simulink model "tricopter_simulation"  (Simulink 7.8)
settings: Solver=FixedStepDiscrete  StartTime=0.0  StopTime=10  FixedStep=dt_sim  RelTol=1e-3
InitFcn:
  | Init
values from neighbouring files (symbols this model uses):
  act_latency = 1*dt_sim    (= 0.005)    [Init.m]
  D = 1    [Init.m]
  dt_sim = 0.005    [Init.m]
  gvec = [0 0 9.81]'    [Init.m]
  J = diag([0.25*m*(D/2)^2 0.25*m*(D/2)^2 0.5*m*(D/2)^2])    [Init.m]
  k = 0.0000192    (= 1.92e-05)    [Init.m]
  L = 0.5    [Init.m]
  m = 1    [Init.m]
  max_rpm = 7000*pi/30    (= 733.038285838)    [Init.m]
  min_rpm = 0    [Init.m]
  rho = 1.26    [Init.m]
undefined symbols (not defined in the file or in its folder): DiscIntNeverNeededParam, waitfortreal
libraries: animation_lib x1, simulink x1
(part 1 of 2)
settings Model: Creator=sven  LastModifiedBy=sven  BufferReuse=off
settings DataIOCC: LimitDataPoints=off  SaveOutput=off  SignalLogging=off  DSMLogging=off  SaveTime=off  SignalLoggingName=sigsOut
settings OptimizationCC: InlineParams=on  BufferReuse=off  InitFltsAndDblsToZero=on
settings DebuggingCC: ConsistencyChecking=error  SignalInfNanChecking=error  SignalRangeChecking=error  ReadBeforeWriteMsg=DisableAll  WriteAfterWriteMsg=DisableAll  WriteAfterReadMsg=DisableAll  AlgebraicLoopMsg=error  ArtificialAlgebraicLoopMsg=error  SaveWithDisabledLinksMsg=error  SaveWithParameterizedLinksMsg=error  UnderspecifiedInitializationDetection=Simplified  MergeDetectMultiDrivingBlocksExec=error  BlockPriorityViolationMsg=error  MinStepSizeMsg=error  TimeAdjustmentMsg=warning  SolverPrmCheckMsg=error  InheritedTsInSrcMsg=error  DiscreteInheritContinuousMsg=error  SingleTaskRateTransMsg=error  TasksWithSamePriorityMsg=error  SigSpecEnsureSampleTimeMsg=error  CheckMatrixSingularityMsg=error  IntegerOverflowMsg=error  ParameterUnderflowMsg=error  ParameterPrecisionLossMsg=error  ParameterTunabilityLossMsg=error  FixptConstUnderflowMsg=error  FixptConstOverflowMsg=error  FixptConstPrecisionLossMsg=error  UnderSpecifiedDataTypeMsg=error  SignalLabelMismatchMsg=error  UnconnectedInputMsg=error  UnconnectedOutputMsg=error  UnconnectedLineMsg=error  SFcnCompatibilityMsg=warning  UniqueDataStoreMsg=error  BusObjectLabelMismatch=error  RootOutportRequireBusObject=error  AssertControl=EnableAll  ModelReferenceIOMsg=error  ModelReferenceVersionMismatchMessage=error  ModelReferenceIOMismatchMessage=error  ModelReferenceCSMismatchMessage=error  UnknownTsInhSupMsg=error  ModelReferenceDataLoggingMessage=error  SimStateInterfaceChecksumMismatchMsg=error  StrictBusMsg=ErrorOnBusTreatedAsVector  BusNameAdapt=ErrorWithoutRepair  NonBusSignalsTreatedAsBus=error  SFUnusedDataAndEventsDiag=error  SFUnexpectedBacktrackingDiag=error  SFInvalidInputDataAccessInChartInitDiag=error  SFNoUnconditionalDefaultTransitionDiag=error  SFTransitionOutsideNaturalParentDiag=error
settings HardwareCC: TargetUnknown=on
settings RTWCC: IncludeERTFirstTime=on
settings GRTTargetCC: TargetFcnLib=ansi_tfl_tmw.mat

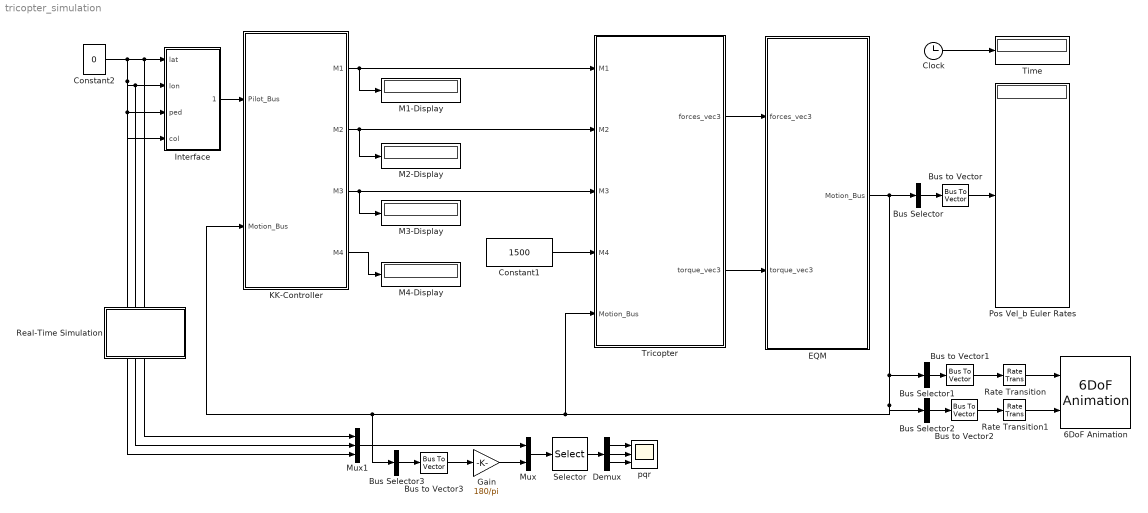
== system tricopter_simulation ==
  6DoF Animation : animation_lib/6DoF Animation  u1=[0 40 -20 20 -50 -30]  u2=0.1  u3=1.0  u4=[40 0 -50]  u5=Fixed position  u6=[20 5 -31]  u7=10  u8=on
  Bus Selector : BusSelector  OutputSignals=pos.x,pos.y,pos.z,vel_body.ub,vel_body.vb,vel_body.wb,attitude.phi,attitude.theta,attitude.psi,rate.p,rate.q,rate.r  OutputAsBus=on
  Bus Selector1 : BusSelector  OutputSignals=pos.x,pos.y,pos.z  OutputAsBus=on
  Bus Selector2 : BusSelector  OutputSignals=attitude.phi,attitude.theta,attitude.psi  OutputAsBus=on
  Bus Selector3 : BusSelector  OutputSignals=rate.p,rate.q,rate.r  OutputAsBus=on
  Bus to Vector{,1..3} (4 alike) : BusToVector
  Clock : Clock
  Constant1 : Constant  Value=1500
  Constant2 : Constant  Value=0
  Demux : Demux  Outputs=3
  EQM : Subsystem
  Gain : Gain  Gain=180/pi
  Interface : Subsystem
  KK-Controller : Subsystem
  M1-Display : Display
  M2-Display : Display
  M3-Display : Display
  M4-Display : Display
  Mux : Mux  Inputs=2
  Mux1 : Mux  Inputs=3
  Pos Vel_b Euler Rates : Display
  Rate Transition : RateTransition  OutPortSampleTime=0.2
  Rate Transition1 : RateTransition  OutPortSampleTime=0.2
  Real-Time Simulation : Subsystem
      mask Display: disp('SL RT')
  Selector : Selector  InputPortWidth=6  IndexOptions=Index vector (dialog)  Indices=[1 4 2 5 3 6]  OutputSizes=1
  Time : Display
  Tricopter : Subsystem
  pqr : Scope  NumInputPorts=3
      settings: YMin=-5~-4~-5  YMax=10~0~5
  wires:
  Tricopter/2(torque_vec3) -> EQM/2(torque_vec3)
  Tricopter/1(forces_vec3) -> EQM/1(forces_vec3)
  EQM/1(Motion_Bus) -> Bus Selector/1, Bus Selector1/1, Tricopter/5(Motion_Bus), KK-Controller/2(Motion_Bus), Bus Selector3/1, Bus Selector2/1
  Constant1/1 -> Tricopter/4(M4)
  KK-Controller/1(M1) -> M1-Display/1, Tricopter/1(M1)
  KK-Controller/2(M2) -> M2-Display/1, Tricopter/2(M2)
  KK-Controller/3(M3) -> M3-Display/1, Tricopter/3(M3)
  Interface/1(Pilot_Bus) -> KK-Controller/1(Pilot_Bus)
  KK-Controller/4(M4) -> M4-Display/1
  Bus Selector/1 -> Bus to Vector/1
  Bus to Vector/1 -> Pos Vel_b Euler Rates/1
  Clock/1 -> Time/1
  Constant2/1 -> Interface/3(ped), Interface/4(col), Mux1/3, Interface/2(lon), Mux1/2, Interface/1(lat), Mux1/1
  Bus Selector1/1 -> Bus to Vector1/1
  Bus Selector2/1 -> Bus to Vector2/1
  Bus to Vector1/1 -> Rate Transition/1
  Bus to Vector2/1 -> Rate Transition1/1
  Rate Transition/1 -> 6DoF Animation/1
  Rate Transition1/1 -> 6DoF Animation/2
  Mux/1 -> Selector/1
  Bus Selector3/1 -> Bus to Vector3/1
  Gain/1 -> Mux/2
  Mux1/1 -> Mux/1
  Selector/1 -> Demux/1
  Demux/1 -> pqr/1
  Demux/2 -> pqr/2
  Demux/3 -> pqr/3
  Bus to Vector3/1 -> Gain/1

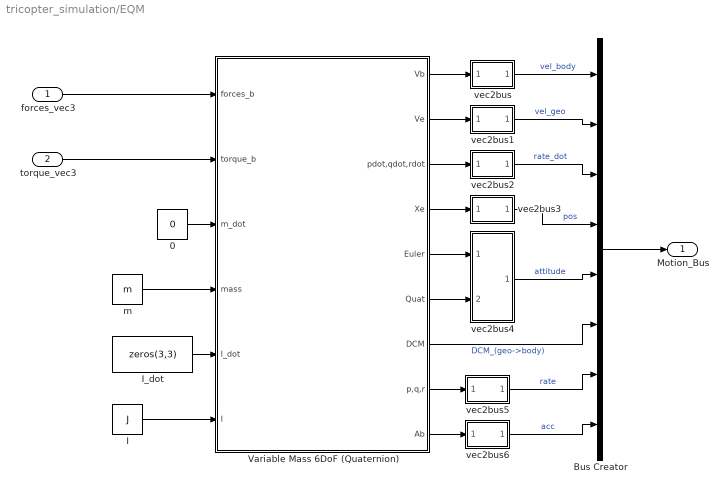
== system tricopter_simulation/EQM ==
  forces_vec3 : Inport
  torque_vec3 : Inport  Port=2
  0 : Constant  Value=0
  Bus Creator : BusCreator  Inputs=8
  I : Constant  Value=J
  I_dot : Constant  Value=zeros(3,3)
  Variable Mass 6DoF (Quaternion) : Subsystem  mask{xme_0=[0 0 0], Vm_0=[0 0 0], eul_0=[0 0 0], pm_0=[10 0 0]*pi/180, dt_sim=dt_sim, run_translation=off}
      mask prompts: xme_0 "Inertial position in inertial axes [Xe, Ye Ze]"; Vm_0 "Inertial velocity in body axes [u, v, w]"; eul_0 "Inertial Euler orientation [roll, pitch, yaw]"; pm_0 "Inertial body rotation rates[p, q, r]"; dt_sim "Sample Time"; run_translation "Run Translational Motion"
      mask help:
      | Variable Mass 6DoF (Quaternion)
      | (rebuild from MATLAB AeroSpace Blockset)
      mask Help:
      | Inputs and Outputs
      | 
      | The first input to the block is a vector containing the three applied forces.
      | The second input is a vector containing the three applied moments.
      | The third input is a scalar containing the rate of change of mass.
      | The fourth input is a scalar containing the mass
      | The fifth input is a 3-by-3 matrix for the rate of change of inertia tensor matrix.
      | The sixth input is a 3-by-3 matrix for the inertia tensor matrix.
      | 
      | The first output is a three-element vector containing the velocity in the Earth-fixed reference frame.
      | The second output is a three-element vector containing the position in the Earth-fixed reference frame.
      | The third output is a three-element vector containing the Euler rotation angles [roll, pitch, yaw], in radians.
      | The fourth output is a 3-by-3 matrix for the coordinate transformation from Earth-fixed axes to body-fixed axes.
      | The fifth output is a three-element vector containing the velocity in the body-fixed frame.
      | The sixth output is a three-element vector containing the angular rates in body-fixed axes, in radians per second.
      | The seventh output is a three-element vector containing the angular accelerations in body-fixed axes, in radians per second. The eighth output is a three-element vector containing the accelerations in body-fixed axes.
      mask Display:
      | port_label('input',1,'Fb_xyz (N)')
      | port_label('input',2,'Mb_xyz (Nm)')
      | port_label('input',3,'dm/dt (kg/s)')
      | port_label('input',4,'m (kg)')
      | port_label('input',5,'dI/dt (kgm^2/s)')
      | port_label('input',6,'I (kgm^2)')
      | port_label('output',1,'Vb (m/s)')
      | port_label('output',2,'Ve (m/s)')
      | port_label('output',3,'pqrdot')
      | port_label('output',4,'Xe')
      | port_label('output',5,'phi theta psi (rad)')
      | port_label('output',6,'quaternions')
      | port_label('output',7,'DCM')
      | port_label('output',8,'pqr')
      | port_label('output',9,'Ab (m/s^2)')
  m : Constant  Value=m
  vec2bus : Subsystem
  vec2bus1 : Subsystem
  vec2bus2 : Subsystem
  vec2bus3 : Subsystem
  vec2bus4 : Subsystem
  vec2bus5 : Subsystem
  vec2bus6 : Subsystem
  Motion_Bus : Outport
  wires:
  vec2bus6/1(bus) -> Bus Creator/8  "acc"
  vec2bus5/1(bus) -> Bus Creator/7  "rate"
  Variable Mass 6DoF (Quaternion)/7(DCM) -> Bus Creator/6  "DCM_(geo->body)"
  vec2bus4/1(bus) -> Bus Creator/5  "attitude"
  vec2bus3/1(bus) -> Bus Creator/4  "pos"
  vec2bus2/1(bus) -> Bus Creator/3  "rate_dot"
  vec2bus1/1(bus) -> Bus Creator/2  "vel_geo"
  vec2bus/1(bus) -> Bus Creator/1  "vel_body"
  Variable Mass 6DoF (Quaternion)/6(Quat) -> vec2bus4/2(quat)
  Variable Mass 6DoF (Quaternion)/9(Ab) -> vec2bus6/1(vec)
  Variable Mass 6DoF (Quaternion)/8(p,q,r) -> vec2bus5/1(vec)
  Variable Mass 6DoF (Quaternion)/5(Euler) -> vec2bus4/1(euler)
  Variable Mass 6DoF (Quaternion)/4(Xe) -> vec2bus3/1(vec)
  Variable Mass 6DoF (Quaternion)/3(pdot,qdot,rdot) -> vec2bus2/1(vec)
  Variable Mass 6DoF (Quaternion)/2(Ve) -> vec2bus1/1(vec)
  Variable Mass 6DoF (Quaternion)/1(Vb) -> vec2bus/1(vec)
  I/1 -> Variable Mass 6DoF (Quaternion)/6(I)
  I_dot/1 -> Variable Mass 6DoF (Quaternion)/5(I_dot)
  m/1 -> Variable Mass 6DoF (Quaternion)/4(mass)
  0/1 -> Variable Mass 6DoF (Quaternion)/3(m_dot)
  forces_vec3/1 -> Variable Mass 6DoF (Quaternion)/1(forces_b)
  torque_vec3/1 -> Variable Mass 6DoF (Quaternion)/2(torque_b)
  Bus Creator/1 -> Motion_Bus/1

== system tricopter_simulation/Interface ==
  lat : Inport
  lon : Inport  Port=2
  ped : Inport  Port=3
  col : Inport  Port=4
  Bus Creator : BusCreator
  Constant1 : Constant  Value=1500
  Demux : Demux
  Display : Display
  Gain1 : Gain  Gain=-1  Multiplication=Matrix(K*u)  SaturateOnIntegerOverflow=on  OutDataTypeStr=Inherit: Same as input  ParamDataTypeStr=Inherit: Same as input
  Gain2 : Gain  Gain=500  Multiplication=Matrix(K*u)  SaturateOnIntegerOverflow=on  OutDataTypeStr=Inherit: Same as input  ParamDataTypeStr=Inherit: Same as input
  Mux2 : Mux
  Sum1 : Sum  SaturateOnIntegerOverflow=on
  Pilot_Bus : Outport
  wires:
  Mux2/1 -> Gain2/1
  lat/1 -> Mux2/1
  lon/1 -> Mux2/2
  ped/1 -> Mux2/3
  col/1 -> Gain1/1
  Constant1/1 -> Sum1/2
  Gain2/1 -> Sum1/1
  Gain1/1 -> Mux2/4
  Sum1/1 -> Demux/1, Display/1
  Demux/1 -> Bus Creator/1  "lat_us"
  Demux/2 -> Bus Creator/2  "lon_us"
  Demux/3 -> Bus Creator/3  "ped_us"
  Demux/4 -> Bus Creator/4  "col_us"
  Bus Creator/1 -> Pilot_Bus/1  "Pilot"

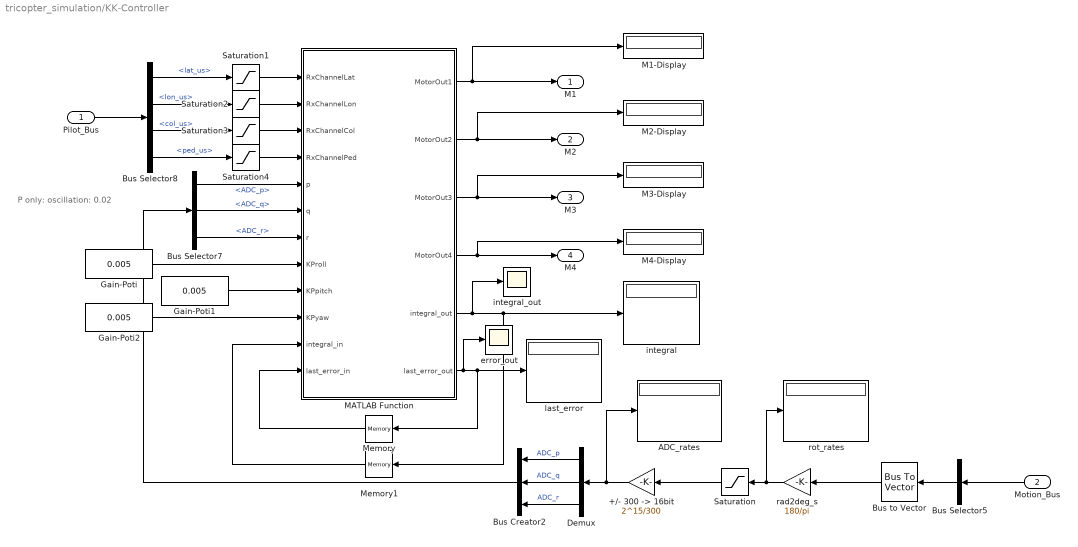
== system tricopter_simulation/KK-Controller ==
  note: P only: oscillation: 0.02
  Pilot_Bus : Inport
  Motion_Bus : Inport  Port=2
  "+/- 300 -> 16bit" : Gain  Gain=2^15/300
  ADC_rates : Display
  Bus Creator2 : BusCreator  Inputs=3
  Bus Selector5 : BusSelector  OutputSignals=rate.p,rate.q,rate.r  OutputAsBus=on
  Bus Selector7 : BusSelector  OutputSignals=ADC_p,ADC_q,ADC_r
  Bus Selector8 : BusSelector  OutputSignals=lat_us,lon_us,col_us,ped_us
  Bus to Vector : BusToVector
  Demux : Demux  Outputs=3
  Gain-Poti : Constant  Value=0.005
  Gain-Poti1 : Constant  Value=0.005
  Gain-Poti2 : Constant  Value=0.005
  M1-Display : Display
  M2-Display : Display
  M3-Display : Display
  M4-Display : Display
  MATLAB Function : MATLAB Function  TreatAsAtomicUnit=on
  Memory : Memory
  Memory1 : Memory
  Saturation : Saturate  UpperLimit=300  LowerLimit=-300
  Saturation{1..4} (4 alike) : Saturate  UpperLimit=2000  LowerLimit=1000
  error_out : Scope
      settings: YMin=-5.5  YMax=1  SaveName=ScopeData3
  integral : Display
  integral_out : Scope
      settings: TimeRange=10  YMin=-50  YMax=50  SaveName=ScopeData2
  last_error : Display
  rad2deg_s : Gain  Gain=180/pi
  rot_rates : Display
  M1 : Outport
  M2 : Outport  Port=2
  M3 : Outport  Port=3
  M4 : Outport  Port=4
  wires:
  MATLAB Function/1(MotorOut1) -> M1-Display/1, M1/1
  MATLAB Function/2(MotorOut2) -> M2-Display/1, M2/1
  MATLAB Function/3(MotorOut3) -> M3-Display/1, M3/1
  Bus Selector5/1 -> Bus to Vector/1
  rad2deg_s/1 -> Saturation/1, rot_rates/1
  Saturation/1 -> "+/- 300 -> 16bit"/1
  "+/- 300 -> 16bit"/1 -> Demux/1, ADC_rates/1
  Demux/1 -> Bus Creator2/1  "ADC_p"
  Demux/2 -> Bus Creator2/2  "ADC_q"
  Demux/3 -> Bus Creator2/3  "ADC_r"
  Bus Creator2/1 -> Bus Selector7/1
  Bus Selector7/1 -> MATLAB Function/5(p)  "<ADC_p>"
  Bus Selector7/2 -> MATLAB Function/6(q)  "<ADC_q>"
  Bus Selector7/3 -> MATLAB Function/7(r)  "<ADC_r>"
  MATLAB Function/4(MotorOut4) -> M4-Display/1, M4/1
  Bus to Vector/1 -> rad2deg_s/1
  Bus Selector8/1 -> Saturation1/1  "<lat_us>"
  Bus Selector8/2 -> Saturation2/1  "<lon_us>"
  Bus Selector8/3 -> Saturation3/1  "<col_us>"
  Bus Selector8/4 -> Saturation4/1  "<ped_us>"
  Saturation1/1 -> MATLAB Function/1(RxChannelLat)
  Saturation2/1 -> MATLAB Function/2(RxChannelLon)
  Saturation3/1 -> MATLAB Function/3(RxChannelCol)
  Saturation4/1 -> MATLAB Function/4(RxChannelPed)
  MATLAB Function/6(last_error_out) -> last_error/1, Memory/1, error_out/1
  MATLAB Function/5(integral_out) -> integral/1, Memory1/1, integral_out/1
  Memory/1 -> MATLAB Function/12(last_error_in)
  Memory1/1 -> MATLAB Function/11(integral_in)
  Motion_Bus/1 -> Bus Selector5/1
  Pilot_Bus/1 -> Bus Selector8/1
  Gain-Poti/1 -> MATLAB Function/8(KProll)
  Gain-Poti1/1 -> MATLAB Function/9(KPpitch)
  Gain-Poti2/1 -> MATLAB Function/10(KPyaw)

== system tricopter_simulation/Real-Time Simulation ==
  Clock : Clock
  MATLAB Fcn : MATLABFcn  MATLABFcn=waitfortreal(u)  OutputDimensions=0
  wires:
  Clock/1 -> MATLAB Fcn/1

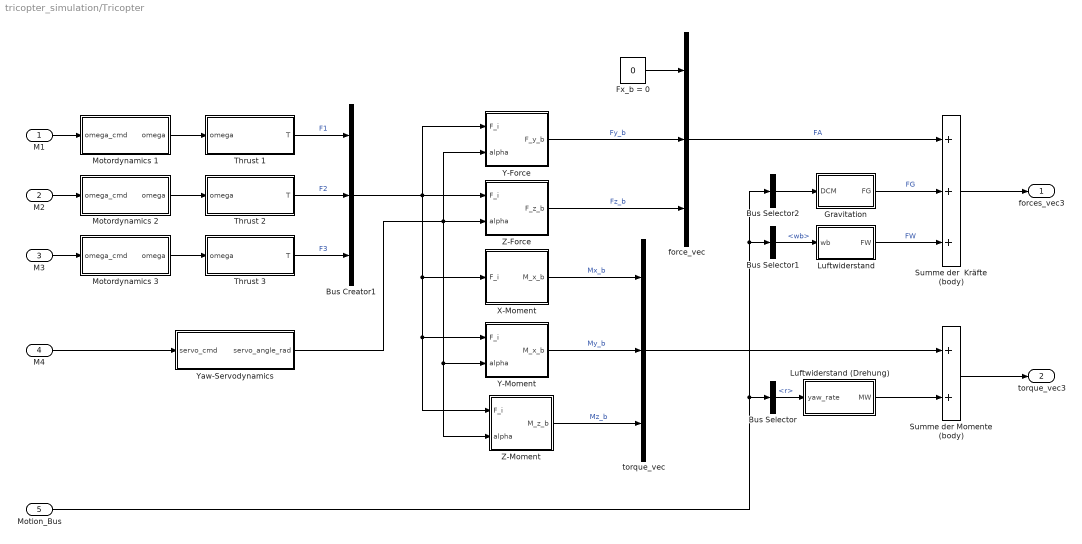
== system tricopter_simulation/Tricopter ==
  M1 : Inport
  M2 : Inport  Port=2
  M3 : Inport  Port=3
  M4 : Inport  Port=4
  Motion_Bus : Inport  Port=5
  Bus Creator1 : BusCreator  Inputs=3
  Bus Selector : BusSelector  OutputSignals=rate.r
  Bus Selector1 : BusSelector  OutputSignals=vel_body.wb
  Bus Selector2 : BusSelector  OutputSignals=DCM_(geo->body)  OutputAsBus=on
  Fx_b = 0 : Constant  Value=0
  Gravitation : Subsystem
  Luftwiderstand : Subsystem
  Luftwiderstand (Drehung) : Subsystem
  Motordynamics 1 : Subsystem
  Motordynamics 2 : Subsystem
  Motordynamics 3 : Subsystem
  Summe der  Kräfte (body) : Sum  Inputs=+++  SaturateOnIntegerOverflow=on
  Summe der Momente (body) : Sum  SaturateOnIntegerOverflow=on
  Thrust 1 : Subsystem
  Thrust 2 : Subsystem
  Thrust 3 : Subsystem
  X-Moment : Subsystem
  Y-Force : Subsystem
  Y-Moment : Subsystem
  Yaw-Servodynamics : Subsystem
  Z-Force : Subsystem
  Z-Moment : Subsystem
  force_vec : Mux  Inputs=3
  torque_vec : Mux  Inputs=3
  forces_vec3 : Outport
  torque_vec3 : Outport  Port=2
  wires:
  Motordynamics 1/1(omega) -> Thrust 1/1(omega)
  Summe der Momente (body)/1 -> torque_vec3/1
  Summe der  Kräfte (body)/1 -> forces_vec3/1
  Bus Selector2/1 -> Gravitation/1(DCM)
  Bus Selector1/1 -> Luftwiderstand/1(wb)  "<wb>"
  Bus Selector/1 -> Luftwiderstand (Drehung)/1(yaw_rate)  "<r>"
  Z-Moment/1(M_z_b) -> torque_vec/3  "Mz_b"
  Luftwiderstand (Drehung)/1(MW) -> Summe der Momente (body)/2
  torque_vec/1 -> Summe der Momente (body)/1
  Luftwiderstand/1(FW) -> Summe der  Kräfte (body)/3  "FW"
  X-Moment/1(M_x_b) -> torque_vec/1  "Mx_b"
  force_vec/1 -> Summe der  Kräfte (body)/1  "FA"
  Z-Force/1(F_z_b) -> force_vec/3  "Fz_b"
  Gravitation/1(FG) -> Summe der  Kräfte (body)/2  "FG"
  Motordynamics 2/1(omega) -> Thrust 2/1(omega)
  Motordynamics 3/1(omega) -> Thrust 3/1(omega)
  Thrust 1/1(T) -> Bus Creator1/1  "F1"
  Thrust 2/1(T) -> Bus Creator1/2  "F2"
  Thrust 3/1(T) -> Bus Creator1/3  "F3"
  Yaw-Servodynamics/1(servo_angle_rad) -> Z-Force/2(alpha), Y-Force/2(alpha), Y-Moment/2(alpha), Z-Moment/2(alpha)
  Bus Creator1/1 -> Z-Force/1(F_i), Y-Force/1(F_i), X-Moment/1(F_i), Y-Moment/1(F_i), Z-Moment/1(F_i)
  Y-Force/1(F_y_b) -> force_vec/2  "Fy_b"
  Fx_b = 0/1 -> force_vec/1
  Y-Moment/1(M_x_b) -> torque_vec/2  "My_b"
  M1/1 -> Motordynamics 1/1(omega_cmd)
  M2/1 -> Motordynamics 2/1(omega_cmd)
  M3/1 -> Motordynamics 3/1(omega_cmd)
  Motion_Bus/1 -> Bus Selector/1, Bus Selector1/1, Bus Selector2/1
  M4/1 -> Yaw-Servodynamics/1(servo_cmd)

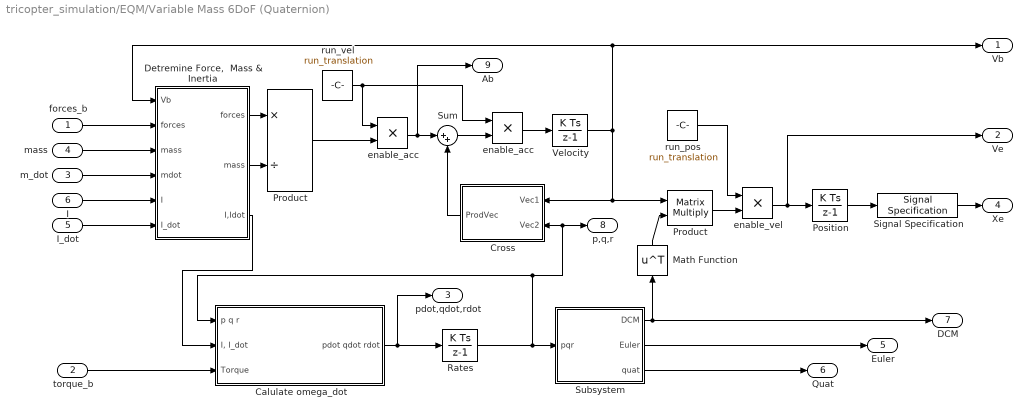
== system tricopter_simulation/EQM/Variable Mass 6DoF (Quaternion) ==
  forces_b : Inport
  torque_b : Inport  Port=2
  m_dot : Inport  Port=3
  mass : Inport  Port=4
  I_dot : Inport  Port=5
  I : Inport  Port=6
  Calulate omega_dot : Subsystem
  Cross : Subsystem
  "Detremine Force,  Mass & Inertia" : Subsystem
  Math Function : Math  Operator=transpose  SaturateOnIntegerOverflow=on
  Position : DiscreteIntegrator  InitialCondition=xme_0  SampleTime=dt_sim  ICPrevOutput=DiscIntNeverNeededParam  ICPrevScaledInput=DiscIntNeverNeededParam
  Product : Product  Inputs=*/  SaturateOnIntegerOverflow=on  OutDataTypeStr=Inherit: Same as first input
  "Product " : Product  Multiplication=Matrix(*)  SaturateOnIntegerOverflow=on  OutDataTypeStr=Inherit: Same as first input
  Rates : DiscreteIntegrator  InitialCondition=pm_0  SampleTime=dt_sim  ICPrevOutput=DiscIntNeverNeededParam  ICPrevScaledInput=DiscIntNeverNeededParam
  Signal Specification : SignalSpecification  OutDataTypeStr=double
  Subsystem : Subsystem
  Sum : Sum  Inputs=|++  SaturateOnIntegerOverflow=on
  Velocity : DiscreteIntegrator  InitialCondition=Vm_0  SampleTime=dt_sim  ICPrevOutput=DiscIntNeverNeededParam  ICPrevScaledInput=DiscIntNeverNeededParam
  enable_acc : Product  RndMeth=Zero
  "enable_acc " : Product  RndMeth=Zero
  enable_vel : Product  RndMeth=Zero
  run_pos : Constant  Value=run_translation  OutMin=0  OutMax=1
  run_vel : Constant  Value=run_translation  OutMin=0  OutMax=1
  Vb : Outport
  Ve : Outport  Port=2
  pdot,qdot,rdot : Outport  Port=3
  Xe : Outport  Port=4
  Euler : Outport  Port=5
  Quat : Outport  Port=6
  DCM : Outport  Port=7
  p,q,r : Outport  Port=8
  Ab : Outport  Port=9
  wires:
  Subsystem/2(Euler) -> Euler/1
  Position/1 -> Signal Specification/1
  enable_vel/1 -> Ve/1, Position/1
  "Detremine Force,  Mass & Inertia"/3(I,Idot) -> Calulate omega_dot/2("I, I_dot")
  torque_b/1 -> Calulate omega_dot/3(Torque)
  Calulate omega_dot/1(pdot qdot rdot) -> pdot,qdot,rdot/1, Rates/1
  Rates/1 -> Calulate omega_dot/1(p q r), Cross/2(Vec2), p,q,r/1, Subsystem/1(pqr)
  Subsystem/1(DCM) -> DCM/1, Math Function/1
  Math Function/1 -> "Product "/2
  Cross/1(ProdVec) -> Sum/2
  Sum/1 -> enable_acc/2
  Velocity/1 -> Vb/1, "Detremine Force,  Mass & Inertia"/1(Vb), Cross/1(Vec1), "Product "/1
  "Detremine Force,  Mass & Inertia"/2("mass ") -> Product/2
  "Detremine Force,  Mass & Inertia"/1("forces ") -> Product/1
  I_dot/1 -> "Detremine Force,  Mass & Inertia"/6(I_dot)
  I/1 -> "Detremine Force,  Mass & Inertia"/5(I)
  m_dot/1 -> "Detremine Force,  Mass & Inertia"/4(mdot)
  mass/1 -> "Detremine Force,  Mass & Inertia"/3(mass)
  forces_b/1 -> "Detremine Force,  Mass & Inertia"/2(forces)
  Subsystem/3(quat) -> Quat/1
  Signal Specification/1 -> Xe/1
  run_pos/1 -> enable_vel/1
  "Product "/1 -> enable_vel/2
  run_vel/1 -> "enable_acc "/1, enable_acc/1
  "enable_acc "/1 -> Ab/1, Sum/1
  Product/1 -> "enable_acc "/2
  enable_acc/1 -> Velocity/1

== system tricopter_simulation/EQM/vec2bus ==
  vec : Inport
  Bus Creator : BusCreator  Inputs=3
  Demux : Demux  Outputs=3
  bus : Outport
  wires:
  Demux/1 -> Bus Creator/1  "ub"
  Demux/2 -> Bus Creator/2  "vb"
  Demux/3 -> Bus Creator/3  "wb"
  Bus Creator/1 -> bus/1
  vec/1 -> Demux/1

== system tricopter_simulation/EQM/vec2bus1 ==
  vec : Inport
  Bus Creator : BusCreator  Inputs=3
  Demux : Demux  Outputs=3
  bus : Outport
  wires:
  vec/1 -> Demux/1
  Bus Creator/1 -> bus/1
  Demux/3 -> Bus Creator/3  "wg"
  Demux/2 -> Bus Creator/2  "vg"
  Demux/1 -> Bus Creator/1  "ug"

== system tricopter_simulation/EQM/vec2bus2 ==
  vec : Inport
  Bus Creator : BusCreator  Inputs=3
  Demux : Demux  Outputs=3
  bus : Outport
  wires:
  Demux/1 -> Bus Creator/1  "pdot"
  Demux/2 -> Bus Creator/2  "qdot"
  Demux/3 -> Bus Creator/3  "rdot"
  Bus Creator/1 -> bus/1
  vec/1 -> Demux/1

== system tricopter_simulation/EQM/vec2bus3 ==
  vec : Inport
  Bus Creator : BusCreator  Inputs=3
  Demux : Demux  Outputs=3
  bus : Outport
  wires:
  vec/1 -> Demux/1
  Bus Creator/1 -> bus/1
  Demux/3 -> Bus Creator/3  "z"
  Demux/2 -> Bus Creator/2  "y"
  Demux/1 -> Bus Creator/1  "x"

== system tricopter_simulation/EQM/vec2bus4 ==
  euler : Inport
  quat : Inport  Port=2
  Bus Creator : BusCreator  Inputs=7
  Demux : Demux  Outputs=3
  Demux1 : Demux
  bus : Outport
  wires:
  Demux/1 -> Bus Creator/1  "phi"
  Demux/2 -> Bus Creator/2  "theta"
  Demux/3 -> Bus Creator/3  "psi"
  Demux1/1 -> Bus Creator/4  "q0"
  Demux1/2 -> Bus Creator/5  "q1"
  Demux1/3 -> Bus Creator/6  "q2"
  Demux1/4 -> Bus Creator/7  "q3"
  euler/1 -> Demux/1
  Bus Creator/1 -> bus/1
  quat/1 -> Demux1/1

== system tricopter_simulation/EQM/vec2bus5 ==
  vec : Inport
  Bus Creator : BusCreator  Inputs=3
  Demux : Demux  Outputs=3
  bus : Outport
  wires:
  vec/1 -> Demux/1
  Bus Creator/1 -> bus/1
  Demux/3 -> Bus Creator/3  "r"
  Demux/2 -> Bus Creator/2  "q"
  Demux/1 -> Bus Creator/1  "p"

== system tricopter_simulation/EQM/vec2bus6 ==
  vec : Inport
  Bus Creator : BusCreator  Inputs=3
  Demux : Demux  Outputs=3
  bus : Outport
  wires:
  Demux/1 -> Bus Creator/1  "ax"
  Demux/2 -> Bus Creator/2  "ay"
  Demux/3 -> Bus Creator/3  "az"
  Bus Creator/1 -> bus/1
  vec/1 -> Demux/1

== system tricopter_simulation/Tricopter/Gravitation ==
  DCM : Inport
  G : Constant  Value=gvec*m
  T_i->b : Product  Multiplication=Matrix(*)  SaturateOnIntegerOverflow=on  OutDataTypeStr=Inherit: Same as first input
  FG : Outport
  wires:
  G/1 -> T_i->b/2
  DCM/1 -> T_i->b/1
  T_i->b/1 -> FG/1

== system tricopter_simulation/Tricopter/Luftwiderstand ==
  wb : Inport
  0 : Constant  Value=0
  A=pi*r^2 : Constant  Value=pi*(D/2)^2
  Direction : Gain  Gain=-1  SaturateOnIntegerOverflow=on  OutDataTypeStr=Inherit: Same as input  ParamDataTypeStr=Inherit: Same as input
  G : Constant  Value=rho/2
  Mux : Mux  Inputs=3
  Sign : Signum
  V^2 : Product  SaturateOnIntegerOverflow=on  OutDataTypeStr=Inherit: Same as first input
  Wz : Product  Inputs=4  SaturateOnIntegerOverflow=on  OutDataTypeStr=Inherit: Same as first input
  FW : Outport
  wires:
  G/1 -> Wz/2
  wb/1 -> V^2/1, V^2/2, Sign/1
  V^2/1 -> Wz/1
  A=pi*r^2/1 -> Wz/3
  Wz/1 -> Mux/3
  Mux/1 -> FW/1
  0/1 -> Mux/1, Mux/2
  Sign/1 -> Direction/1
  Direction/1 -> Wz/4

== system tricopter_simulation/Tricopter/Luftwiderstand (Drehung) ==
  yaw_rate : Inport
  0 : Constant  Value=0
  A=pi*r^2 : Constant  Value=3e-4
  Direction : Gain  Gain=-1  SaturateOnIntegerOverflow=on  OutDataTypeStr=Inherit: Same as input  ParamDataTypeStr=Inherit: Same as input
  Mr : Product  Inputs=3  SaturateOnIntegerOverflow=on  OutDataTypeStr=Inherit: Same as first input
  Mux : Mux  Inputs=3
  Sign : Signum
  r^2 : Product  SaturateOnIntegerOverflow=on  OutDataTypeStr=Inherit: Same as first input
  MW : Outport
  wires:
  Direction/1 -> Mr/3
  Sign/1 -> Direction/1
  0/1 -> Mux/2, Mux/1
  Mux/1 -> MW/1
  Mr/1 -> Mux/3
  A=pi*r^2/1 -> Mr/2
  r^2/1 -> Mr/1
  yaw_rate/1 -> Sign/1, r^2/2, r^2/1

== system tricopter_simulation/Tricopter/Motordynamics 1 ==
  note: DC Motor Dynamics are still missing!
  omega_cmd : Inport
  1-D Lookup Table : Lookup_n-D  NumberOfTableDimensions=1  BreakpointsForDimension1=[900 2100]  Table=[0 7000]*pi/30  RndMeth=Simplest  InputSameDT=on
  Delay : Delay  DelayLength=act_latency/dt_sim  InitialCondition=1
  Mux : Mux  Inputs=2
  "Nonlinear Actuator (Second Order, discrete)" : Subsystem  mask(Second Order Nonlinear Actuator ){wn_fin=17, z_fin=0.95, fin_max=max_rpm, fin_min=min_rpm, fin_maxrate=inf, fin_act_0=[0], offset=0, dt_act=dt_sim}
      mask prompts: wn_fin "Natural frequency:"; z_fin "Damping ratio:"; fin_max "Maximum deflection:"; fin_min "Minimum deflection:"; fin_maxrate "Maximum rate:"; fin_act_0 "Initial position:"; dt_act "SampleTime"
      mask help: Implement a second-order actuator model with saturation and rate limits.
      mask Help: web(asbhelp);
      mask Display:
      | port_label('input',1,'A_{demand}','texmode','on');
      | port_label('output',1,'A_{actual}','texmode','on');
  Scope : Scope
  omega : Outport
  wires:
  omega_cmd/1 -> 1-D Lookup Table/1
  1-D Lookup Table/1 -> Delay/1
  Delay/1 -> "Nonlinear Actuator (Second Order, discrete)"/1(Ac_dem), Mux/1
  "Nonlinear Actuator (Second Order, discrete)"/1(Ac_ac) -> omega/1, Mux/2
  Mux/1 -> Scope/1

== system tricopter_simulation/Tricopter/Motordynamics 2 ==
  note: DC Motor Dynamics are still missing!
  omega_cmd : Inport
  1-D Lookup Table : Lookup_n-D  NumberOfTableDimensions=1  BreakpointsForDimension1=[900 2100]  Table=[0 7000]*pi/30  RndMeth=Simplest  InputSameDT=on
  Delay : Delay  DelayLength=act_latency/dt_sim  InitialCondition=1
  "Nonlinear Actuator (Second Order, discrete)" : Subsystem  mask(Second Order Nonlinear Actuator ){wn_fin=17, z_fin=0.95, fin_max=max_rpm, fin_min=min_rpm, fin_maxrate=inf, fin_act_0=[0], offset=0, dt_act=dt_sim}
      mask prompts: wn_fin "Natural frequency:"; z_fin "Damping ratio:"; fin_max "Maximum deflection:"; fin_min "Minimum deflection:"; fin_maxrate "Maximum rate:"; fin_act_0 "Initial position:"; dt_act "SampleTime"
      mask help: Implement a second-order actuator model with saturation and rate limits.
      mask Help: web(asbhelp);
      mask Display:
      | port_label('input',1,'A_{demand}','texmode','on');
      | port_label('output',1,'A_{actual}','texmode','on');
  omega : Outport
  wires:
  "Nonlinear Actuator (Second Order, discrete)"/1(Ac_ac) -> omega/1
  Delay/1 -> "Nonlinear Actuator (Second Order, discrete)"/1(Ac_dem)
  1-D Lookup Table/1 -> Delay/1
  omega_cmd/1 -> 1-D Lookup Table/1

== system tricopter_simulation/Tricopter/Motordynamics 3 ==
  note: DC Motor Dynamics are still missing!
  omega_cmd : Inport
  1-D Lookup Table : Lookup_n-D  NumberOfTableDimensions=1  BreakpointsForDimension1=[900 2100]  Table=[0 7000]*pi/30  RndMeth=Simplest  InputSameDT=on
  Delay : Delay  DelayLength=act_latency/dt_sim  InitialCondition=1
  "Nonlinear Actuator (Second Order, discrete)" : Subsystem  mask(Second Order Nonlinear Actuator ){wn_fin=17, z_fin=0.95, fin_max=max_rpm, fin_min=min_rpm, fin_maxrate=inf, fin_act_0=[0], offset=0, dt_act=dt_sim}
      mask prompts: wn_fin "Natural frequency:"; z_fin "Damping ratio:"; fin_max "Maximum deflection:"; fin_min "Minimum deflection:"; fin_maxrate "Maximum rate:"; fin_act_0 "Initial position:"; dt_act "SampleTime"
      mask help: Implement a second-order actuator model with saturation and rate limits.
      mask Help: web(asbhelp);
      mask Display:
      | port_label('input',1,'A_{demand}','texmode','on');
      | port_label('output',1,'A_{actual}','texmode','on');
  omega : Outport
  wires:
  omega_cmd/1 -> 1-D Lookup Table/1
  1-D Lookup Table/1 -> Delay/1
  Delay/1 -> "Nonlinear Actuator (Second Order, discrete)"/1(Ac_dem)
  "Nonlinear Actuator (Second Order, discrete)"/1(Ac_ac) -> omega/1

== system tricopter_simulation/Tricopter/Thrust 1 ==
  omega : Inport
  Direction : Gain  Gain=-1  SaturateOnIntegerOverflow=on  OutDataTypeStr=Inherit: Same as input  ParamDataTypeStr=Inherit: Same as input
  k : Gain  Gain=k  SaturateOnIntegerOverflow=on  OutDataTypeStr=Inherit: Same as input  ParamDataTypeStr=Inherit: Same as input
  omega^2 : Product  SaturateOnIntegerOverflow=on  OutDataTypeStr=Inherit: Same as first input
  T : Outport
  wires:
  omega/1 -> omega^2/2, omega^2/1
  omega^2/1 -> k/1
  k/1 -> Direction/1
  Direction/1 -> T/1

== system tricopter_simulation/Tricopter/Thrust 2 ==
  omega : Inport
  Direction : Gain  Gain=-1  SaturateOnIntegerOverflow=on  OutDataTypeStr=Inherit: Same as input  ParamDataTypeStr=Inherit: Same as input
  k : Gain  Gain=k  SaturateOnIntegerOverflow=on  OutDataTypeStr=Inherit: Same as input  ParamDataTypeStr=Inherit: Same as input
  omega^2 : Product  SaturateOnIntegerOverflow=on  OutDataTypeStr=Inherit: Same as first input
  T : Outport
  wires:
  Direction/1 -> T/1
  k/1 -> Direction/1
  omega^2/1 -> k/1
  omega/1 -> omega^2/1, omega^2/2

== system tricopter_simulation/Tricopter/Thrust 3 ==
  omega : Inport
  Direction : Gain  Gain=-1  SaturateOnIntegerOverflow=on  OutDataTypeStr=Inherit: Same as input  ParamDataTypeStr=Inherit: Same as input
  k : Gain  Gain=k  SaturateOnIntegerOverflow=on  OutDataTypeStr=Inherit: Same as input  ParamDataTypeStr=Inherit: Same as input
  omega^2 : Product  SaturateOnIntegerOverflow=on  OutDataTypeStr=Inherit: Same as first input
  T : Outport
  wires:
  omega/1 -> omega^2/2, omega^2/1
  omega^2/1 -> k/1
  k/1 -> Direction/1
  Direction/1 -> T/1

== system tricopter_simulation/Tricopter/X-Moment ==
  F_i : Inport
  Add : Sum  Inputs=-+
  Bus Selector5 : BusSelector  OutputSignals=F1
  Bus Selector7 : BusSelector  OutputSignals=F2
  Gain : Gain  Gain=3/2
  Laenge Arm : Constant  Value=L
  Product : Product  RndMeth=Zero
  Sqrt : Sqrt  SaturateOnIntegerOverflow=on
  M_x_b : Outport
  wires:
  Add/1 -> Product/1
  Bus Selector7/1 -> Add/2  "<F2>"
  Bus Selector5/1 -> Add/1  "<F1>"
  F_i/1 -> Bus Selector5/1, Bus Selector7/1
  Laenge Arm/1 -> Gain/1
  Gain/1 -> Sqrt/1
  Product/1 -> M_x_b/1
  Sqrt/1 -> Product/2

== system tricopter_simulation/Tricopter/Y-Force ==
  F_i : Inport
  alpha : Inport  Port=2
  Bus Selector8 : BusSelector  OutputSignals=F3
  Product : Product  RndMeth=Zero
  Trigonometric Function : Trigonometry
  F_y_b : Outport
  wires:
  alpha/1 -> Trigonometric Function/1
  Trigonometric Function/1 -> Product/2
  Product/1 -> F_y_b/1
  Bus Selector8/1 -> Product/1  "<F3>"
  F_i/1 -> Bus Selector8/1

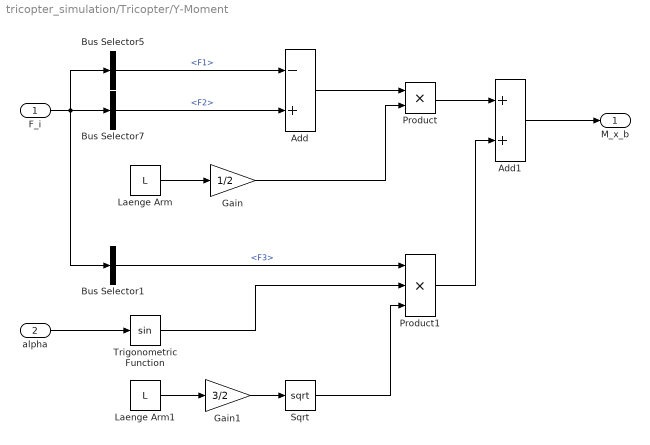
== system tricopter_simulation/Tricopter/Y-Moment ==
  F_i : Inport
  alpha : Inport  Port=2
  Add : Sum  Inputs=-+
  Add1 : Sum
  Bus Selector1 : BusSelector  OutputSignals=F3
  Bus Selector5 : BusSelector  OutputSignals=F1
  Bus Selector7 : BusSelector  OutputSignals=F2
  Gain : Gain  Gain=1/2
  Gain1 : Gain  Gain=3/2
  Laenge Arm : Constant  Value=L
  Laenge Arm1 : Constant  Value=L
  Product : Product  RndMeth=Zero
  Product1 : Product  Inputs=3  RndMeth=Zero
  Sqrt : Sqrt  SaturateOnIntegerOverflow=on
  Trigonometric Function : Trigonometry
  M_x_b : Outport
  wires:
  Product/1 -> Add1/1
  Gain/1 -> Product/2
  Laenge Arm/1 -> Gain/1
  F_i/1 -> Bus Selector7/1, Bus Selector5/1, Bus Selector1/1
  Bus Selector5/1 -> Add/1  "<F1>"
  Bus Selector7/1 -> Add/2  "<F2>"
  Add/1 -> Product/1
  Add1/1 -> M_x_b/1
  Product1/1 -> Add1/2
  Laenge Arm1/1 -> Gain1/1
  Gain1/1 -> Sqrt/1
  Sqrt/1 -> Product1/3
  Bus Selector1/1 -> Product1/1  "<F3>"
  Trigonometric Function/1 -> Product1/2
  alpha/1 -> Trigonometric Function/1

== system tricopter_simulation/Tricopter/Yaw-Servodynamics ==
  servo_cmd : Inport
  1-D Lookup Table : Lookup_n-D  NumberOfTableDimensions=1  BreakpointsForDimension1=[900 2100]  Table=[-60 60]*pi/180  RndMeth=Simplest  InputSameDT=on
  servo_angle_rad : Outport
  wires:
  1-D Lookup Table/1 -> servo_angle_rad/1
  servo_cmd/1 -> 1-D Lookup Table/1

== system tricopter_simulation/Tricopter/Z-Force ==
  F_i : Inport
  alpha : Inport  Port=2
  Add : Sum  Inputs=+++
  Bus Selector5 : BusSelector  OutputSignals=F1
  Bus Selector7 : BusSelector  OutputSignals=F2
  Bus Selector8 : BusSelector  OutputSignals=F3
  Display : Display
  Display1 : Display
  Display2 : Display
  Product : Product  RndMeth=Zero
  Trigonometric Function : Trigonometry  Operator=cos
  F_z_b : Outport
  wires:
  F_i/1 -> Bus Selector8/1, Bus Selector7/1, Bus Selector5/1
  Bus Selector5/1 -> Add/1, Display/1  "<F1>"
  Bus Selector7/1 -> Add/2, Display1/1  "<F2>"
  Bus Selector8/1 -> Product/1  "<F3>"
  Product/1 -> Add/3, Display2/1
  Trigonometric Function/1 -> Product/2
  Add/1 -> F_z_b/1
  alpha/1 -> Trigonometric Function/1

== system tricopter_simulation/Tricopter/Z-Moment ==
  F_i : Inport
  alpha : Inport  Port=2
  Add1 : Sum
  Bus Selector1 : BusSelector  OutputSignals=F3
  Laenge Arm1 : Constant  Value=L
  M_drag : Constant  Value=0
  Product1 : Product  Inputs=3  RndMeth=Zero
  Trigonometric Function : Trigonometry
  M_z_b : Outport
  wires:
  alpha/1 -> Trigonometric Function/1
  Trigonometric Function/1 -> Product1/2
  Bus Selector1/1 -> Product1/1  "<F3>"
  Laenge Arm1/1 -> Product1/3
  Product1/1 -> Add1/2
  Add1/1 -> M_z_b/1
  F_i/1 -> Bus Selector1/1
  M_drag/1 -> Add1/1

== system tricopter_simulation/EQM/Variable Mass 6DoF (Quaternion)/Calulate omega_dot ==
  p q r : Inport
  "I, I_dot" : Inport  Port=2
  Torque : Inport  Port=3
  Cross : Subsystem
  Product : Product  Inputs=/*  Multiplication=Matrix(*)  SaturateOnIntegerOverflow=on  OutDataTypeStr=Inherit: Same as first input
  Reshape : Reshape
  Selector : Selector  NumberOfDimensions=2  InputPortWidth=3  IndexOptions=Index vector (dialog),Select all  Indices=1:3,-1  OutputSizes=1
  Selector1 : Selector  NumberOfDimensions=2  InputPortWidth=3  IndexOptions=Index vector (dialog),Select all  Indices=4:6,-1  OutputSizes=1
  Selector2 : Selector  NumberOfDimensions=2  InputPortWidth=3  IndexOptions=Index vector (dialog),Select all  Indices=1:3,-1  OutputSizes=1
  Subsystem : Subsystem
  Subsystem1 : Subsystem
  Sum : Sum  Inputs=+--  SaturateOnIntegerOverflow=on
  pdot qdot rdot : Outport
  wires:
  Cross/1(ProdVec) -> Sum/3
  Product/1 -> Reshape/1
  Subsystem/1(I*w) -> Cross/2(Vec2)
  Selector2/1 -> Subsystem/2(Inertia)
  p q r/1 -> Subsystem1/2(p q r), Cross/1(Vec1), Subsystem/1(p q r)
  Torque/1 -> Sum/1
  Reshape/1 -> pdot qdot rdot/1
  Sum/1 -> Product/2
  Subsystem1/1(Id*w) -> Sum/2
  Selector1/1 -> Subsystem1/1(I_dot)
  Selector/1 -> Product/1
  "I, I_dot"/1 -> Selector2/1, Selector1/1, Selector/1

== system tricopter_simulation/EQM/Variable Mass 6DoF (Quaternion)/Cross ==
  Vec1 : Inport
  Vec2 : Inport  Port=2
  Product1 : Product  SaturateOnIntegerOverflow=on  InputSameDT=on  OutDataTypeStr=Inherit: Same as first input
  Product2 : Product  SaturateOnIntegerOverflow=on  InputSameDT=on  OutDataTypeStr=Inherit: Same as first input
  Selector : Selector  InputPortWidth=3  IndexOptions=Index vector (dialog)  Indices=[2 3 1]  OutputSizes=1
  Selector1 : Selector  InputPortWidth=3  IndexOptions=Index vector (dialog)  Indices=[3 1 2]  OutputSizes=1
  Selector2 : Selector  InputPortWidth=3  IndexOptions=Index vector (dialog)  Indices=[3 1 2]  OutputSizes=1
  Selector3 : Selector  InputPortWidth=3  IndexOptions=Index vector (dialog)  Indices=[2 3 1]  OutputSizes=1
  Sum1 : Sum  Inputs=+-  SaturateOnIntegerOverflow=on  InputSameDT=on  OutDataTypeStr=Inherit: Same as first input
  ProdVec : Outport
  wires:
  Sum1/1 -> ProdVec/1
  Product2/1 -> Sum1/2
  Product1/1 -> Sum1/1
  Selector3/1 -> Product2/2
  Selector2/1 -> Product2/1
  Selector1/1 -> Product1/2
  Selector/1 -> Product1/1
  Vec2/1 -> Selector1/1, Selector3/1
  Vec1/1 -> Selector/1, Selector2/1

== system tricopter_simulation/EQM/Variable Mass 6DoF (Quaternion)/Detremine Force,  Mass & Inertia ==
  Vb : Inport
  forces : Inport  Port=2
  mass : Inport  Port=3
  mdot : Inport  Port=4
  I : Inport  Port=5
  I_dot : Inport  Port=6
  Matrix Concatenation : Concatenate  Mode=Multidimensional array
  Product : Product  SaturateOnIntegerOverflow=on  OutDataTypeStr=Inherit: Same as first input
  Sum : Sum  Inputs=|++  SaturateOnIntegerOverflow=on
  "forces " : Outport
  "mass " : Outport  Port=2
  I,Idot : Outport  Port=3
  wires:
  Matrix Concatenation/1 -> I,Idot/1
  mass/1 -> "mass "/1
  Sum/1 -> "forces "/1
  forces/1 -> Sum/1
  Vb/1 -> Product/1
  mdot/1 -> Product/2
  I_dot/1 -> Matrix Concatenation/2
  I/1 -> Matrix Concatenation/1
  Product/1 -> Sum/2

== system tricopter_simulation/EQM/Variable Mass 6DoF (Quaternion)/Subsystem ==
  pqr : Inport
  Attitude Reset : Constant  Value=0
  Body Rates Integration : Subsystem  mask{dt_sim=dt_sim}
      mask prompts: dt_sim "Sample Time"
  Initial Euler Angles : Constant  Value=eul_0
  Quadternions to Direct Cosine Matrix : Subsystem
  "Quaternions to Euler Angles " : Subsystem
  euler2quad : Subsystem
  DCM : Outport
  Euler : Outport  Port=2
  quat : Outport  Port=3
  wires:
  "Quaternions to Euler Angles "/1(Euler) -> Euler/1
  Quadternions to Direct Cosine Matrix/1(DCM) -> DCM/1
  Body Rates Integration/1(quaternion) -> Quadternions to Direct Cosine Matrix/1(Quaternions), quat/1, "Quaternions to Euler Angles "/1(Quaternions)
  Initial Euler Angles/1 -> euler2quad/1(Euler)
  pqr/1 -> Body Rates Integration/1(pqr)
  euler2quad/1(Quaternions) -> Body Rates Integration/3(initial_quat)
  Attitude Reset/1 -> Body Rates Integration/2(reset)

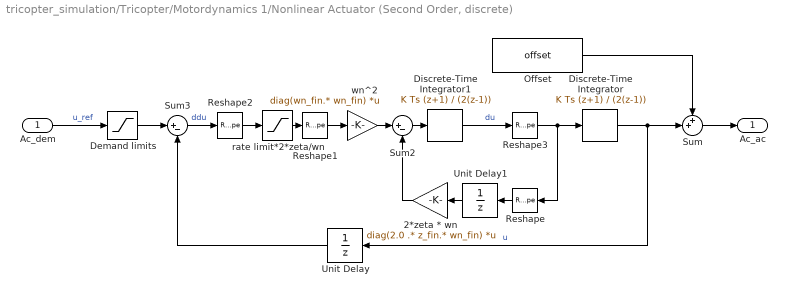
== system tricopter_simulation/Tricopter/Motordynamics 1/Nonlinear Actuator (Second Order, discrete) ==
  Ac_dem : Inport
  2*zeta * wn : Gain  Gain=diag(2.0 .* z_fin.* wn_fin)  Multiplication=Matrix(K*u)  SaturateOnIntegerOverflow=on  OutDataTypeStr=Inherit: Same as input  ParamDataTypeStr=Inherit: Same as input
  Demand limits : Saturate  UpperLimit=fin_max  LowerLimit=fin_min
  Discrete-Time Integrator : DiscreteIntegrator  IntegratorMethod=Integration: Trapezoidal  InitialCondition=fin_act_0  SampleTime=dt_act  LimitOutput=on  UpperSaturationLimit=fin_max  LowerSaturationLimit=fin_min  ICPrevOutput=DiscIntNeverNeededParam  ICPrevScaledInput=DiscIntNeverNeededParam
  Discrete-Time Integrator1 : DiscreteIntegrator  IntegratorMethod=Integration: Trapezoidal  SampleTime=dt_act  ICPrevOutput=DiscIntNeverNeededParam  ICPrevScaledInput=DiscIntNeverNeededParam
  Offset : Constant  Value=offset  SampleTime=dt_act
  Reshape : Reshape  OutputDimensionality=Column vector (2-D)
  Reshape1 : Reshape  OutputDimensionality=Column vector (2-D)
  Reshape2 : Reshape
  Reshape3 : Reshape
  Sum : Sum  Inputs=++|
  Sum2 : Sum  Inputs=|+-  SaturateOnIntegerOverflow=on  InputSameDT=on  OutDataTypeStr=Inherit: Same as first input
  Sum3 : Sum  Inputs=|+-  SaturateOnIntegerOverflow=on  InputSameDT=on  OutDataTypeStr=Inherit: Same as first input
  Unit Delay : UnitDelay  X0=fin_act_0  SampleTime=dt_act
  Unit Delay1 : UnitDelay  SampleTime=dt_act
  rate limit*2*zeta/wn : Saturate  UpperLimit=fin_maxrate.*2.*z_fin./wn_fin  LowerLimit=-fin_maxrate.*2.*z_fin./wn_fin
  wn^2 : Gain  Gain=diag(wn_fin.* wn_fin)  Multiplication=Matrix(K*u)  SaturateOnIntegerOverflow=on  OutDataTypeStr=Inherit: Same as input  ParamDataTypeStr=Inherit: Same as input
  Ac_ac : Outport  InitialOutput=0
  wires:
  Unit Delay/1 -> Sum3/2
  Ac_dem/1 -> Demand limits/1  "u_ref"
  Demand limits/1 -> Sum3/1
  rate limit*2*zeta/wn/1 -> Reshape1/1
  Sum3/1 -> Reshape2/1  "ddu"
  2*zeta * wn/1 -> Sum2/2
  Discrete-Time Integrator1/1 -> Reshape3/1  "du"
  Sum2/1 -> Discrete-Time Integrator1/1
  wn^2/1 -> Sum2/1
  Discrete-Time Integrator/1 -> Unit Delay/1, Sum/2  "u"
  Offset/1 -> Sum/1
  Sum/1 -> Ac_ac/1
  Reshape/1 -> Unit Delay1/1
  Reshape1/1 -> wn^2/1
  Reshape2/1 -> rate limit*2*zeta/wn/1
  Reshape3/1 -> Reshape/1, Discrete-Time Integrator/1
  Unit Delay1/1 -> 2*zeta * wn/1

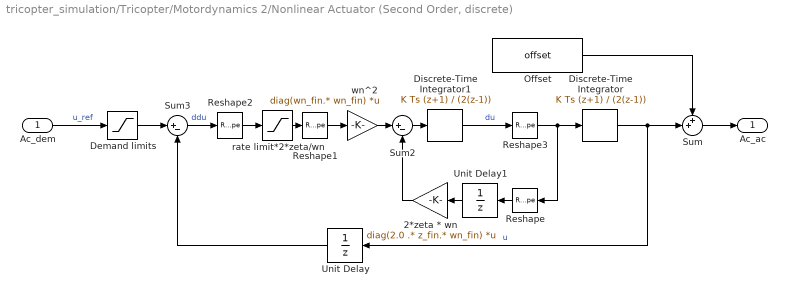
== system tricopter_simulation/Tricopter/Motordynamics 2/Nonlinear Actuator (Second Order, discrete) ==
  Ac_dem : Inport
  2*zeta * wn : Gain  Gain=diag(2.0 .* z_fin.* wn_fin)  Multiplication=Matrix(K*u)  SaturateOnIntegerOverflow=on  OutDataTypeStr=Inherit: Same as input  ParamDataTypeStr=Inherit: Same as input
  Demand limits : Saturate  UpperLimit=fin_max  LowerLimit=fin_min
  Discrete-Time Integrator : DiscreteIntegrator  IntegratorMethod=Integration: Trapezoidal  InitialCondition=fin_act_0  SampleTime=dt_act  LimitOutput=on  UpperSaturationLimit=fin_max  LowerSaturationLimit=fin_min  ICPrevOutput=DiscIntNeverNeededParam  ICPrevScaledInput=DiscIntNeverNeededParam
  Discrete-Time Integrator1 : DiscreteIntegrator  IntegratorMethod=Integration: Trapezoidal  SampleTime=dt_act  ICPrevOutput=DiscIntNeverNeededParam  ICPrevScaledInput=DiscIntNeverNeededParam
  Offset : Constant  Value=offset  SampleTime=dt_act
  Reshape : Reshape  OutputDimensionality=Column vector (2-D)
  Reshape1 : Reshape  OutputDimensionality=Column vector (2-D)
  Reshape2 : Reshape
  Reshape3 : Reshape
  Sum : Sum  Inputs=++|
  Sum2 : Sum  Inputs=|+-  SaturateOnIntegerOverflow=on  InputSameDT=on  OutDataTypeStr=Inherit: Same as first input
  Sum3 : Sum  Inputs=|+-  SaturateOnIntegerOverflow=on  InputSameDT=on  OutDataTypeStr=Inherit: Same as first input
  Unit Delay : UnitDelay  X0=fin_act_0  SampleTime=dt_act
  Unit Delay1 : UnitDelay  SampleTime=dt_act
  rate limit*2*zeta/wn : Saturate  UpperLimit=fin_maxrate.*2.*z_fin./wn_fin  LowerLimit=-fin_maxrate.*2.*z_fin./wn_fin
  wn^2 : Gain  Gain=diag(wn_fin.* wn_fin)  Multiplication=Matrix(K*u)  SaturateOnIntegerOverflow=on  OutDataTypeStr=Inherit: Same as input  ParamDataTypeStr=Inherit: Same as input
  Ac_ac : Outport  InitialOutput=0
  wires:
  Unit Delay1/1 -> 2*zeta * wn/1
  Reshape3/1 -> Discrete-Time Integrator/1, Reshape/1
  Reshape2/1 -> rate limit*2*zeta/wn/1
  Reshape1/1 -> wn^2/1
  Reshape/1 -> Unit Delay1/1
  Sum/1 -> Ac_ac/1
  Offset/1 -> Sum/1
  Discrete-Time Integrator/1 -> Sum/2, Unit Delay/1  "u"
  wn^2/1 -> Sum2/1
  Sum2/1 -> Discrete-Time Integrator1/1
  Discrete-Time Integrator1/1 -> Reshape3/1  "du"
  2*zeta * wn/1 -> Sum2/2
  Sum3/1 -> Reshape2/1  "ddu"
  rate limit*2*zeta/wn/1 -> Reshape1/1
  Demand limits/1 -> Sum3/1
  Ac_dem/1 -> Demand limits/1  "u_ref"
  Unit Delay/1 -> Sum3/2

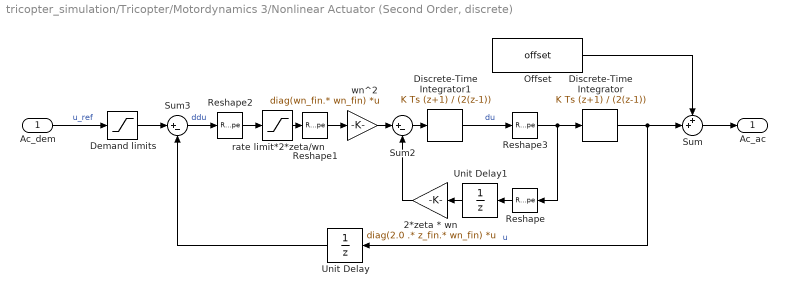
== system tricopter_simulation/Tricopter/Motordynamics 3/Nonlinear Actuator (Second Order, discrete) ==
  Ac_dem : Inport
  2*zeta * wn : Gain  Gain=diag(2.0 .* z_fin.* wn_fin)  Multiplication=Matrix(K*u)  SaturateOnIntegerOverflow=on  OutDataTypeStr=Inherit: Same as input  ParamDataTypeStr=Inherit: Same as input
  Demand limits : Saturate  UpperLimit=fin_max  LowerLimit=fin_min
  Discrete-Time Integrator : DiscreteIntegrator  IntegratorMethod=Integration: Trapezoidal  InitialCondition=fin_act_0  SampleTime=dt_act  LimitOutput=on  UpperSaturationLimit=fin_max  LowerSaturationLimit=fin_min  ICPrevOutput=DiscIntNeverNeededParam  ICPrevScaledInput=DiscIntNeverNeededParam
  Discrete-Time Integrator1 : DiscreteIntegrator  IntegratorMethod=Integration: Trapezoidal  SampleTime=dt_act  ICPrevOutput=DiscIntNeverNeededParam  ICPrevScaledInput=DiscIntNeverNeededParam
  Offset : Constant  Value=offset  SampleTime=dt_act
  Reshape : Reshape  OutputDimensionality=Column vector (2-D)
  Reshape1 : Reshape  OutputDimensionality=Column vector (2-D)
  Reshape2 : Reshape
  Reshape3 : Reshape
  Sum : Sum  Inputs=++|
  Sum2 : Sum  Inputs=|+-  SaturateOnIntegerOverflow=on  InputSameDT=on  OutDataTypeStr=Inherit: Same as first input
  Sum3 : Sum  Inputs=|+-  SaturateOnIntegerOverflow=on  InputSameDT=on  OutDataTypeStr=Inherit: Same as first input
  Unit Delay : UnitDelay  X0=fin_act_0  SampleTime=dt_act
  Unit Delay1 : UnitDelay  SampleTime=dt_act
  rate limit*2*zeta/wn : Saturate  UpperLimit=fin_maxrate.*2.*z_fin./wn_fin  LowerLimit=-fin_maxrate.*2.*z_fin./wn_fin
  wn^2 : Gain  Gain=diag(wn_fin.* wn_fin)  Multiplication=Matrix(K*u)  SaturateOnIntegerOverflow=on  OutDataTypeStr=Inherit: Same as input  ParamDataTypeStr=Inherit: Same as input
  Ac_ac : Outport  InitialOutput=0
  wires:
  Unit Delay/1 -> Sum3/2
  Ac_dem/1 -> Demand limits/1  "u_ref"
  Demand limits/1 -> Sum3/1
  rate limit*2*zeta/wn/1 -> Reshape1/1
  Sum3/1 -> Reshape2/1  "ddu"
  2*zeta * wn/1 -> Sum2/2
  Discrete-Time Integrator1/1 -> Reshape3/1  "du"
  Sum2/1 -> Discrete-Time Integrator1/1
  wn^2/1 -> Sum2/1
  Discrete-Time Integrator/1 -> Unit Delay/1, Sum/2  "u"
  Offset/1 -> Sum/1
  Sum/1 -> Ac_ac/1
  Reshape/1 -> Unit Delay1/1
  Reshape1/1 -> wn^2/1
  Reshape2/1 -> rate limit*2*zeta/wn/1
  Reshape3/1 -> Reshape/1, Discrete-Time Integrator/1
  Unit Delay1/1 -> 2*zeta * wn/1

== system tricopter_simulation/EQM/Variable Mass 6DoF (Quaternion)/Calulate omega_dot/Cross ==
  Vec1 : Inport
  Vec2 : Inport  Port=2
  Product1 : Product  SaturateOnIntegerOverflow=on  InputSameDT=on  OutDataTypeStr=Inherit: Same as first input
  Product2 : Product  SaturateOnIntegerOverflow=on  InputSameDT=on  OutDataTypeStr=Inherit: Same as first input
  Selector : Selector  InputPortWidth=3  IndexOptions=Index vector (dialog)  Indices=[2 3 1]  OutputSizes=1
  Selector1 : Selector  InputPortWidth=3  IndexOptions=Index vector (dialog)  Indices=[3 1 2]  OutputSizes=1
  Selector2 : Selector  InputPortWidth=3  IndexOptions=Index vector (dialog)  Indices=[3 1 2]  OutputSizes=1
  Selector3 : Selector  InputPortWidth=3  IndexOptions=Index vector (dialog)  Indices=[2 3 1]  OutputSizes=1
  Sum1 : Sum  Inputs=+-  SaturateOnIntegerOverflow=on  InputSameDT=on  OutDataTypeStr=Inherit: Same as first input
  ProdVec : Outport
  wires:
  Sum1/1 -> ProdVec/1
  Product2/1 -> Sum1/2
  Product1/1 -> Sum1/1
  Selector3/1 -> Product2/2
  Selector2/1 -> Product2/1
  Selector1/1 -> Product1/2
  Selector/1 -> Product1/1
  Vec2/1 -> Selector1/1, Selector3/1
  Vec1/1 -> Selector/1, Selector2/1

== system tricopter_simulation/EQM/Variable Mass 6DoF (Quaternion)/Calulate omega_dot/Subsystem ==
  p q r : Inport
  Inertia : Inport  Port=2
  Product2 : Product  Multiplication=Matrix(*)  SaturateOnIntegerOverflow=on  OutDataTypeStr=Inherit: Same as first input
  I*w : Outport
  wires:
  p q r/1 -> Product2/2
  Inertia/1 -> Product2/1
  Product2/1 -> I*w/1

== system tricopter_simulation/EQM/Variable Mass 6DoF (Quaternion)/Calulate omega_dot/Subsystem1 ==
  I_dot : Inport
  p q r : Inport  Port=2
  Product2 : Product  Multiplication=Matrix(*)  SaturateOnIntegerOverflow=on  OutDataTypeStr=Inherit: Same as first input
  Id*w : Outport
  wires:
  I_dot/1 -> Product2/1
  Product2/1 -> Id*w/1
  p q r/1 -> Product2/2

== system tricopter_simulation/EQM/Variable Mass 6DoF (Quaternion)/Subsystem/Body Rates Integration ==
  pqr : Inport
  reset : Inport  Port=2
  initial_quat : Inport  Port=3
  Rate Integration : Subsystem  mask{dt_sim=dt_sim}
      mask prompts: dt_sim "Sample Time"
  Unit Delay Resettable External IC : simulink/Additional Math & Discrete/Additional Discrete/Unit Delay Resettable External IC  tsamp=dt_sim
  quaternion : Outport
  wires:
  initial_quat/1 -> Unit Delay Resettable External IC/3
  pqr/1 -> Rate Integration/1(p q r)
  reset/1 -> Unit Delay Resettable External IC/2
  Unit Delay Resettable External IC/1 -> Rate Integration/2(q0 q1 q2 q3)
  Rate Integration/1(q_prod) -> quaternion/1, Unit Delay Resettable External IC/1  "quat"
